simulink model "Quasi"  (R2019b)
settings: Solver=VariableStepAuto  StartTime=0.0  StopTime=0.1  RelTol=1e-3
libraries: powerlib x9, powerlib_meascontrol x1
settings Model: Creator=Niharika  LastModifiedBy=swaga
settings DataIOCC: ReturnWorkspaceOutputs=off

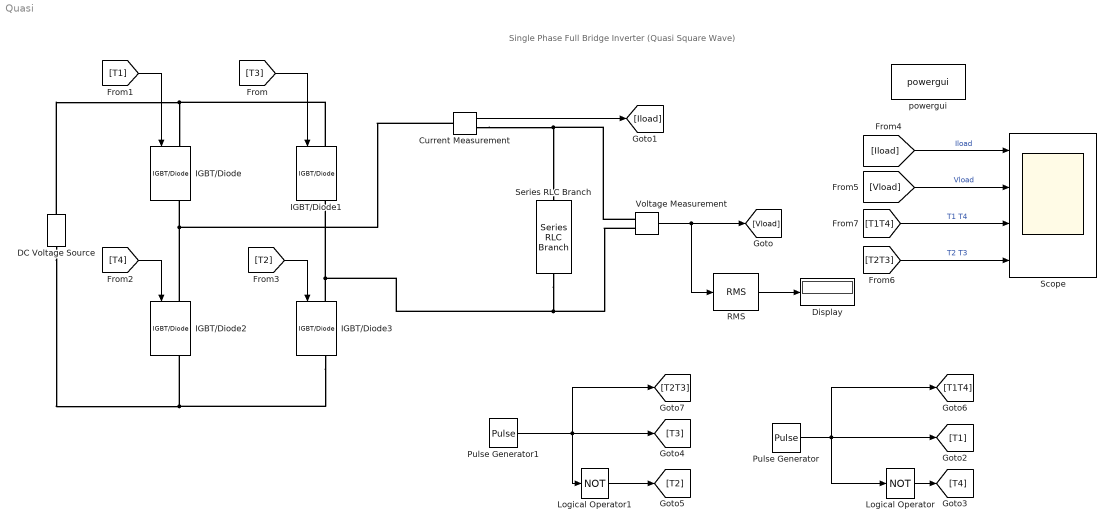
== system Quasi ==
  note: Single Phase Full Bridge Inverter (Quasi Square Wave)
  Current Measurement : powerlib/Measurements/Current Measurement  PhasorSimulation=off  OutputType=Complex  PSBequivalent=0
  DC Voltage Source : powerlib/Electrical Sources/DC Voltage Source  Amplitude=100  Measurements=None
  Display : Display
  IGBT/Diode{,1..3} (4 alike) : powerlib/Power Electronics/IGBT//Diode  Ron=1e-3  Rs=1e5  Cs=inf  Measurements=on
  Logical Operator : Logic  Operator=NOT  AllPortsSameDT=off  OutDataTypeStr=boolean
  Logical Operator1 : Logic  Operator=NOT  AllPortsSameDT=off  OutDataTypeStr=boolean
  Pulse Generator : DiscretePulseGenerator  PulseType=Time based  Period=0.02  PulseWidth=50
  Pulse Generator1 : DiscretePulseGenerator  PulseType=Time based  Period=0.02  PulseWidth=25  PhaseDelay=220/360*0.02
  RMS : powerlib_meascontrol/Measurements/RMS  TrueRMS=on  Freq=60  RMSInit=120  Ts=0
  Scope : Scope  NumInputPorts=4
  Series RLC Branch : powerlib/Elements/Series RLC Branch  LConnTagsString=__new0  RConnTagsString=__new0  BranchType=R  Resistance=10  Inductance=1e-3  SetiL0=off  InitialCurrent=0  Capacitance=1e-6  Setx0=off  InitialVoltage=0  Measurements=Branch voltage and current
  Voltage Measurement : powerlib/Measurements/Voltage Measurement  PhasorSimulation=off  OutputType=Complex  PSBequivalent=0
  powergui : powerlib/powergui  Priority=1  SimulationMode=Discrete  SampleTime=50e-6  frequency=60  Iterations=50  frequencyindice=0  Pbase=100e6  ErrMax=1e-4  UnitsV=kV  UnitsW=MW  buscounter=0  FunctionMessages=off  echomessages=off  EnableUseOfTLC=off  CurrentSourceSwitches=off  DisableSnubberDevices=off  DisableRonSwitches=off  DisableVfSwitches=off  DisplayEquations=off  AutomaticDiscreteSolvers=off  SolverType=Tustin/Backward Euler (TBE)  Interpol=off  ExternalGateDelay=off  methode=off  Ts=100  x0status=blocks  SPID=on  SwTol=0  HookPort=off  NonlinearTolerance=1e-4  nMaxIteration=100  ContinueOnMaxIteration=off  RestoreLinks=warning  ResistiveCurrentMeasurement=off  Frange=[0:2:500]  Ylog=off  Xlog=on  ShowGrid=off  save=off  variable=ZData  structure=SPWM  ZoomFFT=off  StartTime=0.0  cycles=1  DisplayStyle=2  fundamental=50  FreqAxis=off  MaxFrequency=1000  frequencyindicesteady=1  RmsSteady=1  display=off
      settings: SourceProductName=Simscape Electrical
  wires:
  Voltage Measurement/1 -> [Vload], RMS/1
  Current Measurement/1 -> [Iload]
  [T2] -> IGBT/Diode3/1
  [T4] -> IGBT/Diode2/1
  [T1] -> IGBT/Diode/1
  [T3] -> IGBT/Diode1/1
  Logical Operator/1 -> [T4]
  RMS/1 -> Display/1
  [Vload] -> Scope/2  "Vload"
  [Iload] -> Scope/1  "Iload"
  Pulse Generator/1 -> Logical Operator/1, [T1], [T1T4]
  Logical Operator1/1 -> [T2]
  Pulse Generator1/1 -> [T2T3], Logical Operator1/1, [T3]
  [T2T3] -> Scope/4  "T2 T3"
  [T1T4] -> Scope/3  "T1 T4"
  connections:
  IGBT/Diode3/LConn1 -- Voltage Measurement/LConn2 -- Series RLC Branch/RConn1 -- IGBT/Diode1/RConn1
  IGBT/Diode2/LConn1 -- Current Measurement/LConn1 -- IGBT/Diode/RConn1
  DC Voltage Source/LConn1 -- IGBT/Diode2/RConn1 -- IGBT/Diode3/RConn1
  DC Voltage Source/RConn1 -- IGBT/Diode1/LConn1 -- IGBT/Diode/LConn1
  Current Measurement/RConn1 -- Series RLC Branch/LConn1 -- Voltage Measurement/LConn1
